simulink model "Modelo_EQU_tarea2"  (R2024b)
settings: Solver=VariableStepAuto  StartTime=0.0  StopTime=10.0  RelTol=1e-3
undefined symbols (not defined in the file): a, alpha, beta_eq, g_m, gamma, x1_0, x2_0, xr
settings Model: Creator=juanm  LastModifiedBy=juanm

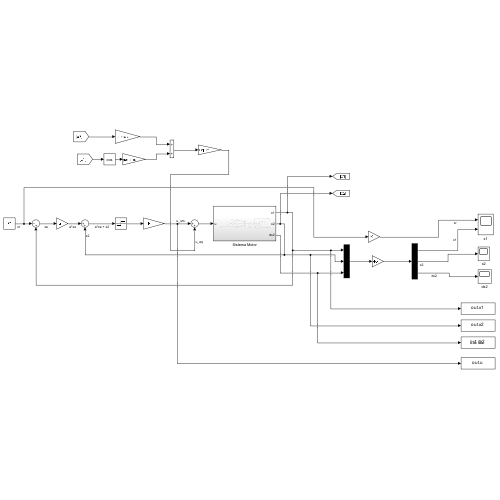
[thumbnail: Simulink's stored preview of the top-level diagram]
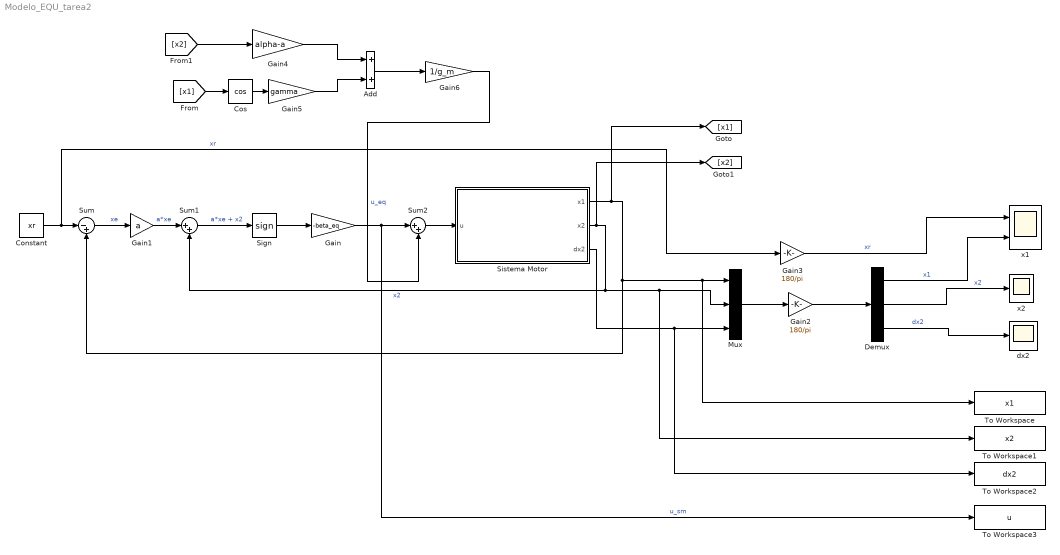
== system Modelo_EQU_tarea2 ==
  Add : Sum
  Constant : Constant  Value=xr
  Cos : Trigonometry  Operator=cos
  Demux : Demux  Outputs=3
  Gain : Gain  Gain=-beta_eq
  Gain1 : Gain  Gain=a
  Gain2 : Gain  Gain=180/pi
  Gain3 : Gain  Gain=180/pi
  Gain4 : Gain  Gain=alpha-a
  Gain5 : Gain  Gain=gamma
  Gain6 : Gain  Gain=1/g_m
  Mux : Mux  Inputs=3
  Sign : Signum  ZeroCross=off
  Sistema Motor : Subsystem
  Sum : Sum  Inputs=|-+
  Sum1 : Sum  Inputs=|++
  Sum2 : Sum  Inputs=|++
  To Workspace : ToWorkspace  VariableName=x1  SaveFormat=Timeseries  SampleTime=-1
  To Workspace1 : ToWorkspace  VariableName=x2  SaveFormat=Timeseries  SampleTime=-1
  To Workspace2 : ToWorkspace  VariableName=dx2  SaveFormat=Timeseries  SampleTime=-1
  To Workspace3 : ToWorkspace  VariableName=u  SaveFormat=Timeseries  SampleTime=-1
  dx2 : Scope
  x1 : Scope  NumInputPorts=2
  x2 : Scope
  wires:
  Constant/1 -> Sum/1, Gain3/1  "xr"
  Demux/2 -> x2/1  "x2"
  Gain3/1 -> x1/1  "xr"
  Sistema Motor/3(dx2) -> To Workspace2/1, Mux/3
  Demux/1 -> x1/2  "x1"
  Gain2/1 -> Demux/1
  Mux/1 -> Gain2/1
  Demux/3 -> dx2/1  "dx2"
  Sum/1 -> Gain1/1  "xe"
  Sign/1 -> Gain/1
  Gain1/1 -> Sum1/1  "a*xe"
  Gain/1 -> Sum2/1, To Workspace3/1  "u_sm"
  Sum1/1 -> Sign/1  "a*xe + x2"
  Sistema Motor/1(x1) -> [x1], To Workspace/1, Mux/1, Sum/2
  Sistema Motor/2(x2) -> [x2], To Workspace1/1, Mux/2, Sum1/2  "x2"
  [x2] -> Gain4/1
  Cos/1 -> Gain5/1
  [x1] -> Cos/1
  Gain4/1 -> Add/1
  Gain5/1 -> Add/2
  Add/1 -> Gain6/1
  Gain6/1 -> Sum2/2  "u_eq"
  Sum2/1 -> Sistema Motor/1(u)

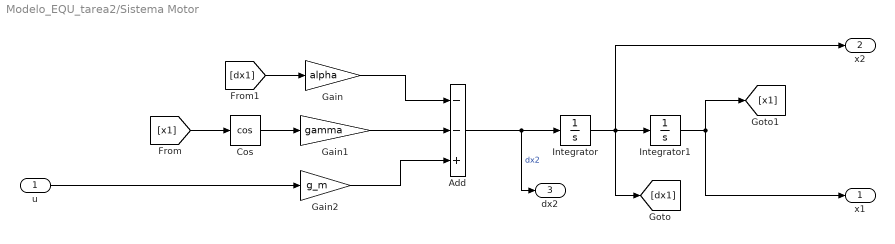
== system Modelo_EQU_tarea2/Sistema Motor ==
  u : Inport
  Add : Sum  Inputs=--+
  Cos : Trigonometry  Operator=cos
  Gain : Gain  Gain=alpha
  Gain1 : Gain  Gain=gamma
  Gain2 : Gain  Gain=g_m
  Integrator : Integrator  InitialCondition=x2_0
  Integrator1 : Integrator  InitialCondition=x1_0
  x1 : Outport
  x2 : Outport  Port=2
  dx2 : Outport  Port=3
  wires:
  Add/1 -> dx2/1, Integrator/1  "dx2"
  Gain1/1 -> Add/2
  Integrator1/1 -> x1/1, [x1]
  Gain2/1 -> Add/3
  Cos/1 -> Gain1/1
  Gain/1 -> Add/1
  Integrator/1 -> x2/1, [dx1], Integrator1/1
  u/1 -> Gain2/1
  [x1] -> Cos/1
  [dx1] -> Gain/1
